simulink model "fxpdemo_direct_form2"  (R2023b)
settings: Solver=FixedStepDiscrete  StartTime=0.0  StopTime=200.0  FixedStep=1  RelTol=1e-3
Description:
  | Fixed-Point Direct Form Filter
  | 
  | This example shows how to implement a direct form filter in fixed point
  | using fundamental building blocks such as Gain, Delay, and Sum.
settings Model: MinMaxOverflowLogging=MinMaxAndOverflow  Creator=The MathWorks, Inc.  LastModifiedBy=amirhossein
settings SolverCC: AlgebraicLoopSolver=TrustRegion  MaxZcPerStep=1
settings DataIOCC: SaveFormat=Array  ReturnWorkspaceOutputs=off  SignalLoggingName=sigsOut
settings OptimizationCC: BooleanDataType=off  ExpressionDepthLimit=2147483647  InitFltsAndDblsToZero=on  LifeSpan=inf
settings DebuggingCC: SaveWithParameterizedLinksMsg=none  UnderspecifiedInitializationDetection=Classic  MergeDetectMultiDrivingBlocksExec=none  SignalResolutionControl=TryResolveAllWithWarning  MultiTaskDSMMsg=warning  MultiTaskCondExecSysMsg=none  IntegerOverflowMsg=none  ParameterDowncastMsg=warning  ParameterOverflowMsg=warning  ParameterPrecisionLossMsg=none  FcnCallInpInsideContextMsg=warning  UnconnectedInputMsg=warning  UnconnectedOutputMsg=warning  UnconnectedLineMsg=warning  StateNameClashWarn=warning  SFUnexpectedBacktrackingDiag=warning  SFNoUnconditionalDefaultTransitionDiag=warning  SFExecutionAtInitializationDiag=none  IntegerSaturationMsg=none  ArithmeticOperatorsInVariantConditions=warning
settings HardwareCC: ProdBitPerPointer=32  ProdBitPerSizeT=32  ProdBitPerPtrDiffT=32  ProdLargestAtomicFloat=None  ProdIntDivRoundTo=Undefined  ProdEndianess=Unspecified  ProdWordSize=32  ProdHWDeviceType=32-bit Generic  TargetUnknown=on
settings ModelReferenceCC: EnableRefExpFcnMdlSchedulingChecks=on  PropagateSignalLabelsOutOfModel=off
settings SFSimCC: SimUseLocalCustomCode=off  CustomCodeUndefinedFunction=UseInterfaceOnly
settings RTWCC: RTWUseLocalCustomCode=off  DLArmComputeVersion=19.05
settings CodeAppCC: StateflowObjectComments=on
settings GRTTargetCC: TargetFcnLib=ansi_tfl_tmw.mat  TargetLangStandard=C89/C90 (ANSI)  CombineOutputUpdateFcns=off  GRTInterface=on
settings ConfigComp: CovMetricSettings=d  CovSaveCumulativeToWorkspaceVar=on  CovSaveSingleToWorkspaceVar=on  CovExternalEMLEnable=off

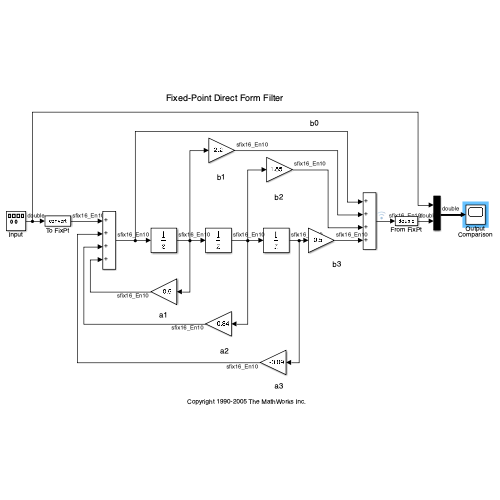
[thumbnail: Simulink's stored preview of the top-level diagram]
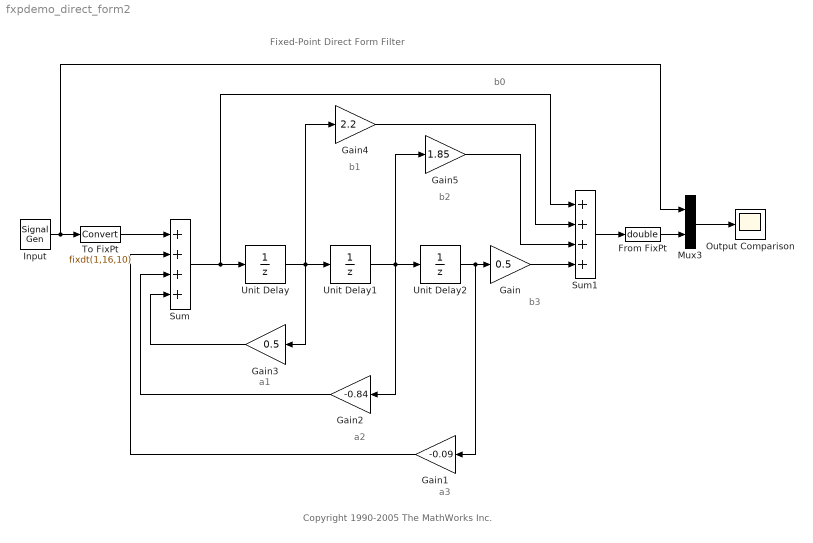
== system fxpdemo_direct_form2 ==
  note: b0
  note: b1
  note: b2
  note: b3
  note: a1
  note: a2
  note: a3
  note: Fixed-Point Direct Form Filter
  note: Copyright 1990-2005 The MathWorks Inc.
  From FixPt : DataTypeConversion  OutDataTypeStr=double  SaturateOnIntegerOverflow=off  RndMeth=Floor
  Gain : Gain  Gain=0.5  ParamDataTypeStr=sfix( 16 )  OutDataTypeStr=fixdt(1,16,10)
  Gain1 : Gain  Gain=-0.09  ParamDataTypeStr=sfix( 16 )  OutDataTypeStr=fixdt(1,16,10)
  Gain2 : Gain  Gain=-0.84  ParamDataTypeStr=sfix( 16 )  OutDataTypeStr=fixdt(1,16,10)
  Gain3 : Gain  Gain=0.5  ParamDataTypeStr=sfix( 16 )  OutDataTypeStr=fixdt(1,16,10)
  Gain4 : Gain  Gain=2.2  ParamDataTypeStr=sfix( 16 )  OutDataTypeStr=fixdt(1,16,10)
  Gain5 : Gain  Gain=1.85  ParamDataTypeStr=sfix( 16 )  OutDataTypeStr=fixdt(1,16,10)
  Input : SignalGenerator  WaveForm=square  Frequency=0.005
  Mux3 : Mux  Inputs=2
  Output Comparison : Scope
  Sum : Sum  Inputs=++++  OutDataTypeStr=fixdt(1,16,10)
  Sum1 : Sum  Inputs=++++  OutDataTypeStr=fixdt(1,16,10)
  To FixPt : DataTypeConversion  OutDataTypeStr=fixdt(1,16,10)  SaturateOnIntegerOverflow=off  RndMeth=Floor
  Unit Delay : UnitDelay  InitialCondition=0.0  SampleTime=1.0  HasFrameUpgradeWarning=on
  Unit Delay1 : UnitDelay  InitialCondition=0.0  SampleTime=1.0  HasFrameUpgradeWarning=on
  Unit Delay2 : UnitDelay  InitialCondition=0.0  SampleTime=1.0  HasFrameUpgradeWarning=on
  wires:
  Input/1 -> Mux3/1, To FixPt/1
  To FixPt/1 -> Sum/1
  Sum/1 -> Sum1/1, Unit Delay/1
  Gain3/1 -> Sum/4
  Unit Delay/1 -> Gain3/1, Gain4/1, Unit Delay1/1
  Gain2/1 -> Sum/3
  Unit Delay1/1 -> Unit Delay2/1, Gain5/1, Gain2/1
  Gain1/1 -> Sum/2
  Gain/1 -> Sum1/4
  Gain5/1 -> Sum1/3
  Gain4/1 -> Sum1/2
  Unit Delay2/1 -> Gain/1, Gain1/1
  Sum1/1 -> From FixPt/1
  From FixPt/1 -> Mux3/2
  Mux3/1 -> Output Comparison/1
